simulink library "Batteries"  (R2025b)
settings: Solver=VariableStepAuto  StartTime=0.0  StopTime=10.0  RelTol=1e-3
undefined symbols (not defined in the file or in its folder): battery_builder_rtmsupport, gcbh
libraries: Batteries_lib x20
(part 2 of 2)

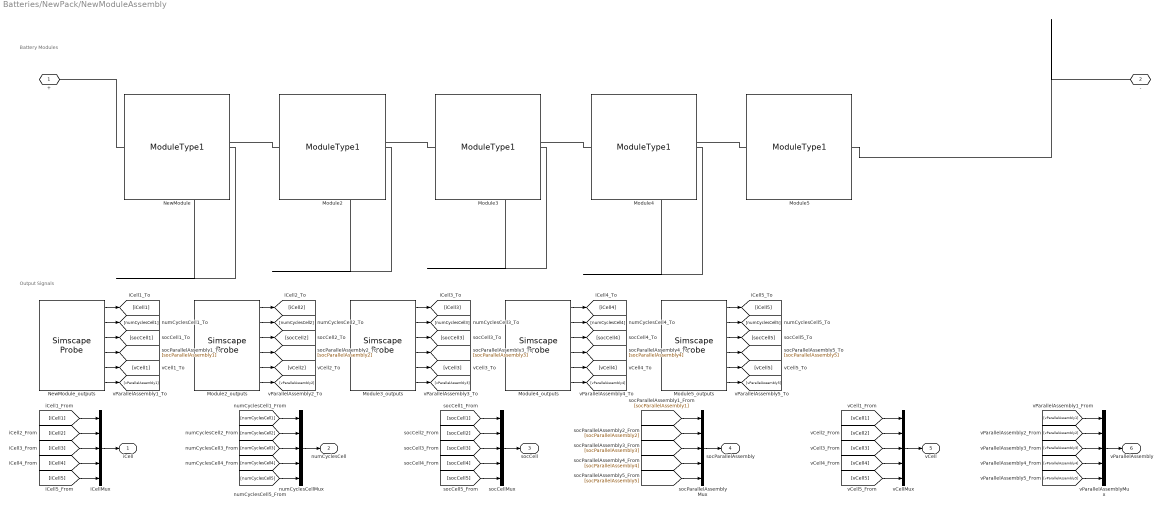
== system Batteries/NewPack/NewModuleAssembly ==
  note: Output Signals
  note: Battery Modules
  Module{2..5} (4 alike) : Batteries_lib/Modules/ModuleType1  SOC_vecCell=[0, .01, .02, .03, .04, .05, .06, .07, .08, .09, .1, .11, .12, .13, .14, .15, .16, .17, .18, .19, .2, .21, .22, .23, .24, .25, .26, .27, .28, .29, .3, .31, .32, .33, .34, .35, .36, .37, .38, .39, .4, .41, .42, .43, .44, .45, .46, .47, .48, .49, .5, .51, .52, .53, .54, .55, .56, .57, .58, .59, .6, .61, .62, .63, .64, .65, .66, .67, .68, .69, .7, .71, .72, .73, .74, .75, .76, .77, .78, .79, .8, .81, .82, .83, .84, .85, .86, .87, .88, .89, .9, .91, .92, .93, .94, .95, .96, .97, .98, .99, 1]  V0_vecCell=[3.17242, 3.18272, 3.19302, 3.20331, 3.21361, 3.22391, 3.23421, 3.24451, 3.25481, 3.2651, 3.2754, 3.2857, 3.296, 3.3063, 3.31659, 3.32689, 3.33719, 3.34749, 3.35779, 3.36809, 3.37838, 3.38868, 3.39898, 3.40928, 3.41958, 3.42988, 3.44017, 3.45047, 3.46077, 3.47107, 3.48137, 3.49166, 3.50196, 3.51226, 3.52256, 3.53286, 3.54316, 3.55345, 3.56375, 3.57405, 3.58435, 3.59465, 3.60495, 3.61524, 3.62554, 3.63584, 3.64614, 3.65644, 3.66673, 3.67703, 3.68733, 3.69763, 3.71041, 3.72113, 3.72997, 3.73882, 3.74912, 3.75936, 3.76951, 3.7791, 3.78865, 3.79787, 3.80709, 3.8161, 3.82509, 3.83409, 3.84308, 3.85207, 3.86107, 3.87006, 3.87901, 3.88831, 3.89824, 3.90887, 3.91951, 3.93012, 3.94073, 3.95138, 3.96184, 3.97226, 3.98268, 3.99311, 4.0032, 4.01221, 4.01944, 4.02668, 4.03286, 4.03874, 4.04383, 4.0488, 4.05377, 4.05873, 4.06312, 4.06753, 4.07333, 4.08117, 4.08904, 4.09911, 4.11111, 4.13802, 4.16831] V  V_rangeCell=[2.25, Inf] V  R0_vecCell=[.02095, .01921, .01774, .0166, .01557, .01469, .01398, .01338, .01283, .01239, .01196, .01155, .01116, .01079, .01042, .01007, .00974, .00949, .00924, .009, .00876, .00855, .00843, .00832, .00826, .00825, .00825, .00826, .00827, .00828, .0083, .00834, .00838, .00842, .00848, .00855, .00863, .00871, .00879, .00887, .00895, .00903, .00911, .00918, .00925, .00931, .00938, .00946, .00953, .00961, .00968, .00976, .00991, .01, .01003, .01006, .01013, .01022, .0103, .01037, .01043, .01049, .01055, .01061, .01066, .01072, .01077, .01082, .01088, .01093, .01099, .01105, .01114, .01125, .01136, .01148, .01161, .01175, .01188, .01202, .01215, .01228, .01241, .01253, .01261, .01269, .01275, .0128, .01285, .01289, .01294, .01298, .01296, .01292, .01292, .01288, .01282, .0128, .01232, .01214, .00952] Ohm  AHCell=4.493 A*hr  extrapolation_optionCell=simscape.enum.extrapolation.nearest  P=1  S=13  iCell_specify=off  iCell_priority=None  iCell=0 A  iCell_nominal_specify=off  iCell_nominal_value=1  iCell_nominal_unit=A  vCell_specify=off  vCell_priority=None  vCell=0 V  vCell_nominal_specify=off  vCell_nominal_value=1  vCell_nominal_unit=V  socCell_specify=off  socCell_priority=High  socCell=1  socCell_nominal_specify=off  socCell_nominal_value=1  socCell_nominal_unit=1  numCyclesCell_specify=off  numCyclesCell_priority=High  numCyclesCell=0  numCyclesCell_nominal_specify=off  numCyclesCell_nominal_value=1  numCyclesCell_nominal_unit=1  vParallelAssembly_specify=off  vParallelAssembly_priority=None  vParallelAssembly=repmat(0, 13, 1) V  vParallelAssembly_nominal_specify=off  vParallelAssembly_nominal_value=1  vParallelAssembly_nominal_unit=V  socParallelAssembly_specify=off  socParallelAssembly_priority=None  socParallelAssembly=repmat(1, 13, 1)  socParallelAssembly_nominal_specify=off  socParallelAssembly_nominal_value=1  socParallelAssembly_nominal_unit=1
      settings: InternalSimscapePortConfiguration="{\"Bottom\":[{\"id\":\"n\",\"label\":\"-\",\"type\":\"foundation.electrical.electrical\"}],\"Left\":[],\"Right\":[],\"Top\":[{\"id\":\"p\",\"label\":\"+\",\"type\":\"foundation.electrical.electrical\"}]}"
  Module2_outputs : SimscapeProbe  BoundBlock=91  Variables="{\"iCell\":{\"Probing\":\"ON\"},\"numCyclesCell\":{\"Probing\":\"ON\"},\"socCell\":{\"Probing\":\"ON\"},\"socParallelAssembly\":{\"Probing\":\"ON\"},\"vCell\":{\"Probing\":\"ON\"},\"vParallelAssembly\":{\"Probing\":\"ON\"}}"
  Module3_outputs : SimscapeProbe  BoundBlock=93  Variables="{\"iCell\":{\"Probing\":\"ON\"},\"numCyclesCell\":{\"Probing\":\"ON\"},\"socCell\":{\"Probing\":\"ON\"},\"socParallelAssembly\":{\"Probing\":\"ON\"},\"vCell\":{\"Probing\":\"ON\"},\"vParallelAssembly\":{\"Probing\":\"ON\"}}"
  Module4_outputs : SimscapeProbe  BoundBlock=95  Variables="{\"iCell\":{\"Probing\":\"ON\"},\"numCyclesCell\":{\"Probing\":\"ON\"},\"socCell\":{\"Probing\":\"ON\"},\"socParallelAssembly\":{\"Probing\":\"ON\"},\"vCell\":{\"Probing\":\"ON\"},\"vParallelAssembly\":{\"Probing\":\"ON\"}}"
  Module5_outputs : SimscapeProbe  BoundBlock=97  Variables="{\"iCell\":{\"Probing\":\"ON\"},\"numCyclesCell\":{\"Probing\":\"ON\"},\"socCell\":{\"Probing\":\"ON\"},\"socParallelAssembly\":{\"Probing\":\"ON\"},\"vCell\":{\"Probing\":\"ON\"},\"vParallelAssembly\":{\"Probing\":\"ON\"}}"
  NewModule : Batteries_lib/Modules/ModuleType1  SOC_vecCell=[0, .01, .02, .03, .04, .05, .06, .07, .08, .09, .1, .11, .12, .13, .14, .15, .16, .17, .18, .19, .2, .21, .22, .23, .24, .25, .26, .27, .28, .29, .3, .31, .32, .33, .34, .35, .36, .37, .38, .39, .4, .41, .42, .43, .44, .45, .46, .47, .48, .49, .5, .51, .52, .53, .54, .55, .56, .57, .58, .59, .6, .61, .62, .63, .64, .65, .66, .67, .68, .69, .7, .71, .72, .73, .74, .75, .76, .77, .78, .79, .8, .81, .82, .83, .84, .85, .86, .87, .88, .89, .9, .91, .92, .93, .94, .95, .96, .97, .98, .99, 1]  V0_vecCell=[3.17242, 3.18272, 3.19302, 3.20331, 3.21361, 3.22391, 3.23421, 3.24451, 3.25481, 3.2651, 3.2754, 3.2857, 3.296, 3.3063, 3.31659, 3.32689, 3.33719, 3.34749, 3.35779, 3.36809, 3.37838, 3.38868, 3.39898, 3.40928, 3.41958, 3.42988, 3.44017, 3.45047, 3.46077, 3.47107, 3.48137, 3.49166, 3.50196, 3.51226, 3.52256, 3.53286, 3.54316, 3.55345, 3.56375, 3.57405, 3.58435, 3.59465, 3.60495, 3.61524, 3.62554, 3.63584, 3.64614, 3.65644, 3.66673, 3.67703, 3.68733, 3.69763, 3.71041, 3.72113, 3.72997, 3.73882, 3.74912, 3.75936, 3.76951, 3.7791, 3.78865, 3.79787, 3.80709, 3.8161, 3.82509, 3.83409, 3.84308, 3.85207, 3.86107, 3.87006, 3.87901, 3.88831, 3.89824, 3.90887, 3.91951, 3.93012, 3.94073, 3.95138, 3.96184, 3.97226, 3.98268, 3.99311, 4.0032, 4.01221, 4.01944, 4.02668, 4.03286, 4.03874, 4.04383, 4.0488, 4.05377, 4.05873, 4.06312, 4.06753, 4.07333, 4.08117, 4.08904, 4.09911, 4.11111, 4.13802, 4.16831] V  V_rangeCell=[2.25, Inf] V  R0_vecCell=[.02095, .01921, .01774, .0166, .01557, .01469, .01398, .01338, .01283, .01239, .01196, .01155, .01116, .01079, .01042, .01007, .00974, .00949, .00924, .009, .00876, .00855, .00843, .00832, .00826, .00825, .00825, .00826, .00827, .00828, .0083, .00834, .00838, .00842, .00848, .00855, .00863, .00871, .00879, .00887, .00895, .00903, .00911, .00918, .00925, .00931, .00938, .00946, .00953, .00961, .00968, .00976, .00991, .01, .01003, .01006, .01013, .01022, .0103, .01037, .01043, .01049, .01055, .01061, .01066, .01072, .01077, .01082, .01088, .01093, .01099, .01105, .01114, .01125, .01136, .01148, .01161, .01175, .01188, .01202, .01215, .01228, .01241, .01253, .01261, .01269, .01275, .0128, .01285, .01289, .01294, .01298, .01296, .01292, .01292, .01288, .01282, .0128, .01232, .01214, .00952] Ohm  AHCell=4.493 A*hr  extrapolation_optionCell=simscape.enum.extrapolation.nearest  P=1  S=13  iCell_specify=off  iCell_priority=None  iCell=0 A  iCell_nominal_specify=off  iCell_nominal_value=1  iCell_nominal_unit=A  vCell_specify=off  vCell_priority=None  vCell=0 V  vCell_nominal_specify=off  vCell_nominal_value=1  vCell_nominal_unit=V  socCell_specify=off  socCell_priority=High  socCell=1  socCell_nominal_specify=off  socCell_nominal_value=1  socCell_nominal_unit=1  numCyclesCell_specify=off  numCyclesCell_priority=High  numCyclesCell=0  numCyclesCell_nominal_specify=off  numCyclesCell_nominal_value=1  numCyclesCell_nominal_unit=1  vParallelAssembly_specify=off  vParallelAssembly_priority=None  vParallelAssembly=repmat(0, 13, 1) V  vParallelAssembly_nominal_specify=off  vParallelAssembly_nominal_value=1  vParallelAssembly_nominal_unit=V  socParallelAssembly_specify=off  socParallelAssembly_priority=None  socParallelAssembly=repmat(1, 13, 1)  socParallelAssembly_nominal_specify=off  socParallelAssembly_nominal_value=1  socParallelAssembly_nominal_unit=1
      settings: InternalSimscapePortConfiguration="{\"Bottom\":[{\"id\":\"n\",\"label\":\"-\",\"type\":\"foundation.electrical.electrical\"}],\"Left\":[],\"Right\":[],\"Top\":[{\"id\":\"p\",\"label\":\"+\",\"type\":\"foundation.electrical.electrical\"}]}"
  NewModule_outputs : SimscapeProbe  BoundBlock=99  Variables="{\"iCell\":{\"Probing\":\"ON\"},\"numCyclesCell\":{\"Probing\":\"ON\"},\"socCell\":{\"Probing\":\"ON\"},\"socParallelAssembly\":{\"Probing\":\"ON\"},\"vCell\":{\"Probing\":\"ON\"},\"vParallelAssembly\":{\"Probing\":\"ON\"}}"
  iCellMux : Mux  Inputs=5
  numCyclesCellMux : Mux  Inputs=5
  socCellMux : Mux  Inputs=5
  socParallelAssemblyMux : Mux  Inputs=5
  vCellMux : Mux  Inputs=5
  vParallelAssemblyMux : Mux  Inputs=5
  + : PMIOPort  Side=Left
  - : PMIOPort  Port=2  Side=Right
  iCell : Outport
  numCyclesCell : Outport  Port=2
  socCell : Outport  Port=3
  socParallelAssembly : Outport  Port=4
  vCell : Outport  Port=5
  vParallelAssembly : Outport  Port=6
  wires:
  [vParallelAssembly5] -> vParallelAssemblyMux/5
  Module5_outputs/6 -> [vParallelAssembly5]
  [vCell5] -> vCellMux/5
  Module5_outputs/5 -> [vCell5]
  [socParallelAssembly5] -> socParallelAssemblyMux/5
  Module5_outputs/4 -> [socParallelAssembly5]
  [socCell5] -> socCellMux/5
  Module5_outputs/3 -> [socCell5]
  [numCyclesCell5] -> numCyclesCellMux/5
  Module5_outputs/2 -> [numCyclesCell5]
  [iCell5] -> iCellMux/5
  Module5_outputs/1 -> [iCell5]
  [vParallelAssembly4] -> vParallelAssemblyMux/4
  Module4_outputs/6 -> [vParallelAssembly4]
  [vCell4] -> vCellMux/4
  Module4_outputs/5 -> [vCell4]
  [socParallelAssembly4] -> socParallelAssemblyMux/4
  Module4_outputs/4 -> [socParallelAssembly4]
  [socCell4] -> socCellMux/4
  Module4_outputs/3 -> [socCell4]
  [numCyclesCell4] -> numCyclesCellMux/4
  Module4_outputs/2 -> [numCyclesCell4]
  [iCell4] -> iCellMux/4
  Module4_outputs/1 -> [iCell4]
  [vParallelAssembly3] -> vParallelAssemblyMux/3
  Module3_outputs/6 -> [vParallelAssembly3]
  [vCell3] -> vCellMux/3
  Module3_outputs/5 -> [vCell3]
  [socParallelAssembly3] -> socParallelAssemblyMux/3
  Module3_outputs/4 -> [socParallelAssembly3]
  [socCell3] -> socCellMux/3
  Module3_outputs/3 -> [socCell3]
  [numCyclesCell3] -> numCyclesCellMux/3
  Module3_outputs/2 -> [numCyclesCell3]
  [iCell3] -> iCellMux/3
  Module3_outputs/1 -> [iCell3]
  [vParallelAssembly2] -> vParallelAssemblyMux/2
  Module2_outputs/6 -> [vParallelAssembly2]
  [vCell2] -> vCellMux/2
  Module2_outputs/5 -> [vCell2]
  [socParallelAssembly2] -> socParallelAssemblyMux/2
  Module2_outputs/4 -> [socParallelAssembly2]
  [socCell2] -> socCellMux/2
  Module2_outputs/3 -> [socCell2]
  [numCyclesCell2] -> numCyclesCellMux/2
  Module2_outputs/2 -> [numCyclesCell2]
  [iCell2] -> iCellMux/2
  Module2_outputs/1 -> [iCell2]
  [vParallelAssembly1] -> vParallelAssemblyMux/1
  vParallelAssemblyMux/1 -> vParallelAssembly/1
  NewModule_outputs/6 -> [vParallelAssembly1]
  [vCell1] -> vCellMux/1
  vCellMux/1 -> vCell/1
  NewModule_outputs/5 -> [vCell1]
  [socParallelAssembly1] -> socParallelAssemblyMux/1
  socParallelAssemblyMux/1 -> socParallelAssembly/1
  NewModule_outputs/4 -> [socParallelAssembly1]
  [socCell1] -> socCellMux/1
  socCellMux/1 -> socCell/1
  NewModule_outputs/3 -> [socCell1]
  [numCyclesCell1] -> numCyclesCellMux/1
  numCyclesCellMux/1 -> numCyclesCell/1
  NewModule_outputs/2 -> [numCyclesCell1]
  [iCell1] -> iCellMux/1
  iCellMux/1 -> iCell/1
  NewModule_outputs/1 -> [iCell1]
  connections:
  Module5/RConn1 -- -/RConn1
  NewModule/LConn1 -- +/RConn1
  Module5/LConn1 -- Module4/RConn1
  Module4/LConn1 -- Module3/RConn1
  Module3/LConn1 -- Module2/RConn1
  Module2/LConn1 -- NewModule/RConn1
